simulink model "PSK"  (R2017a)
settings: Solver=VariableStepAuto  StartTime=0.0  StopTime=10.0  RelTol=1e-3
libraries: commchan3 x1, dsparch4 x1, commrandsrc3 x1, commsink2 x1, dspsigops x1
settings Model: Creator=81228  LastModifiedBy=81228

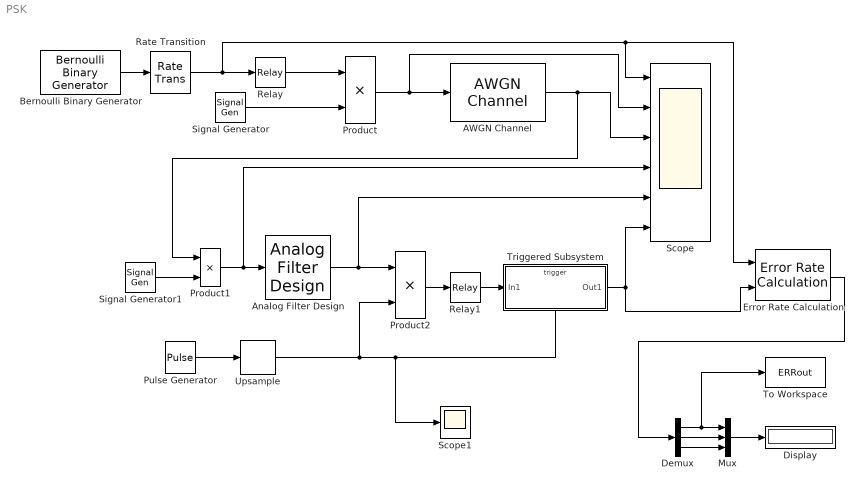
== system PSK ==
  AWGN Channel : commchan3/AWGN Channel  InputProcessing=Columns as channels (frame based)  seed=67  noiseMode=Variance from mask  EbNodB=10  EsNodB=10  SNRdB=10  bitsPerSym=1  Ps=1  Tsym=1  variance=0.2
  Analog Filter Design : dsparch4/Analog Filter Design  method=Butterworth  filttype=Lowpass  N=2  Wlo=8  Whi=80  Rp=2  Rs=40
  Bernoulli Binary Generator : commrandsrc3/Bernoulli Binary Generator  ProbabilityOfZero=0.5  SeedSource=Parameter  Seed=61  SampleTime=1.1  SamplesPerFrame=1  OutputDataType=double  SimulateUsing=Interpreted execution
  Demux : Demux  Outputs=3
  Display : Display
  Error Rate Calculation : commsink2/Error Rate Calculation  N=0  st_delay=0  cp_mode=Entire frame  subframe=[]  PMode=Port  WsName=ErrorVec  RsMode2=off  stop=off  numErr=100  maxBits=1e6
  Mux : Mux  Inputs=3
  Product : Product
  Product1 : Product
  Product2 : Product
  Pulse Generator : DiscretePulseGenerator  Period=50  PulseWidth=50
  Rate Transition : RateTransition  X0=1  OutPortSampleTimeOpt=Multiple of input port sample time
  Relay : Relay  OffOutputValue=-1
  Relay1 : Relay  OffOutputValue=-1
  Scope : Scope  NumInputPorts=6
  Scope1 : Scope
  Signal Generator : SignalGenerator  Amplitude=2  Frequency=4
  Signal Generator1 : SignalGenerator  Amplitude=2  Frequency=4
  To Workspace : ToWorkspace  VariableName=ERRout  SaveFormat=Timeseries  SampleTime=-1
  Triggered Subsystem : Subsystem  TreatAsAtomicUnit=on
  Upsample : dspsigops/Upsample  N=10  phase=0  InputProcessing=Columns as channels (frame based)  RateOptions=Enforce single-rate processing  ic=0  mode=Unused parameter value
  wires:
  Bernoulli Binary Generator/1 -> Rate Transition/1
  Rate Transition/1 -> Scope/1, Error Rate Calculation/1, Relay/1
  Relay/1 -> Product/1
  Signal Generator/1 -> Product/2
  Product/1 -> AWGN Channel/1, Scope/2
  Signal Generator1/1 -> Product1/2
  Product1/1 -> Scope/4, Analog Filter Design/1
  Pulse Generator/1 -> Upsample/1
  Analog Filter Design/1 -> Scope/5, Product2/1
  Upsample/1 -> Scope1/1, Triggered Subsystem/Trigger, Product2/2
  Triggered Subsystem/1(Out1) -> Scope/6, Error Rate Calculation/2
  Relay1/1 -> Triggered Subsystem/1(In1)
  Product2/1 -> Relay1/1
  AWGN Channel/1 -> Product1/1, Scope/3
  Demux/1 -> To Workspace/1, Mux/1
  Demux/2 -> Mux/2
  Demux/3 -> Mux/3
  Error Rate Calculation/1 -> Demux/1
  Mux/1 -> Display/1

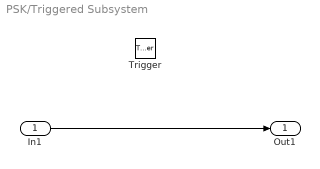
== system PSK/Triggered Subsystem ==
  In1 : Inport
  Trigger : TriggerPort  VariantControl=Variant
  Out1 : Outport
  wires:
  In1/1 -> Out1/1
